simulink model "lab3_main"  (R2023a)
settings: Solver=VariableStepAuto  StartTime=0.0  StopTime=10.0  RelTol=1e-3
model workspace (MAT data in the model file):
  target = 0.05
values from neighbouring files (symbols this model uses):
  anum = 0.3    [lab3.m]
  den = [1 0 w0^2]    [lab3.m]
  denD = cell2mat(denD)    [lab3.m]
  num = G*w0^2    (= 4)    [lab3.m]
  numD = cell2mat(numD)    [lab3.m]
  Ts = 0.1    [lab3.m]
settings Model: Creator=dgkegkas2023  LastModifiedBy=dgkegkas2023

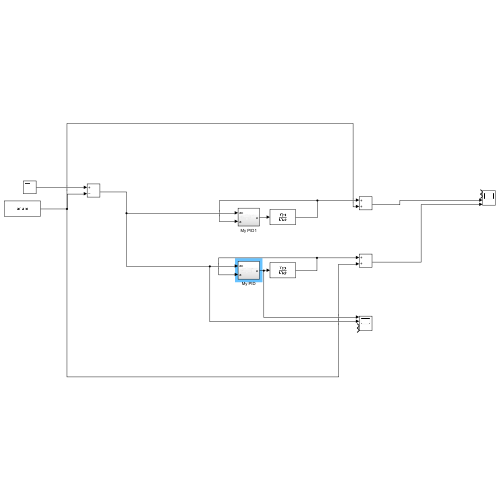
[thumbnail: Simulink's stored preview of the top-level diagram]
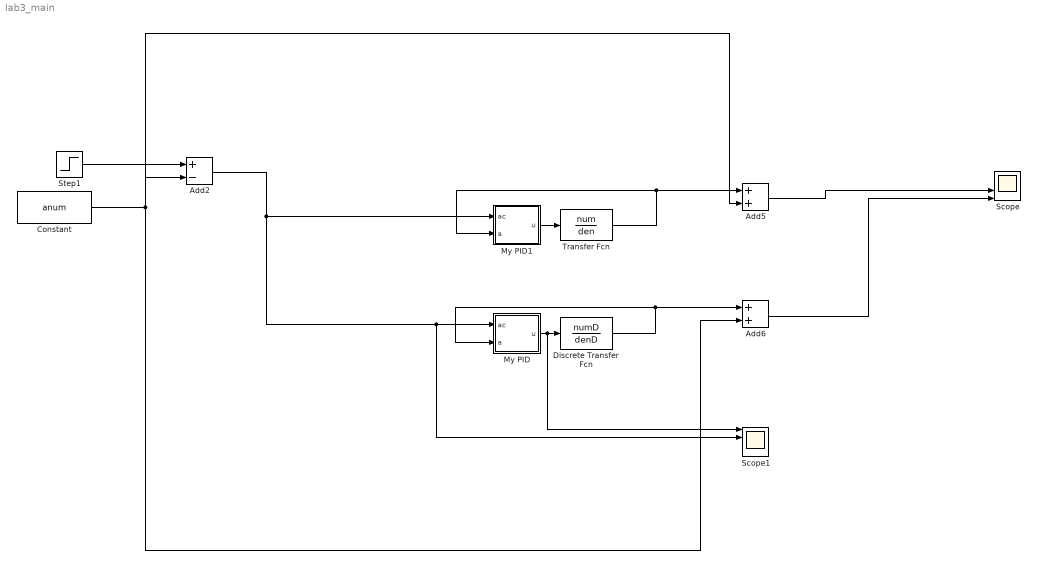
== system lab3_main ==
  Add2 : Sum  Inputs=+-
  Add5 : Sum
  Add6 : Sum
  Constant : Constant  Value=anum
  Discrete Transfer Fcn : DiscreteTransferFcn  Numerator=numD  Denominator=denD
  My PID : Subsystem
  My PID1 : Subsystem
  Scope : Scope  NumInputPorts=4
  Scope1 : Scope  NumInputPorts=4
  Step1 : Step  Before=0.3  After=0.27  SampleTime=Ts
  Transfer Fcn : TransferFcn  Numerator=num  Denominator=den
  wires:
  Transfer Fcn/1 -> My PID1/2(a), Add5/1
  Discrete Transfer Fcn/1 -> My PID/2(a), Add6/1
  Step1/1 -> Add2/1
  Constant/1 -> Add6/2, Add5/2, Add2/2
  Add2/1 -> My PID1/1(ac), Scope1/2, My PID/1(ac)
  Add5/1 -> Scope/3
  Add6/1 -> Scope/4
  My PID1/1(u) -> Transfer Fcn/1
  My PID/1(u) -> Scope1/1, Discrete Transfer Fcn/1

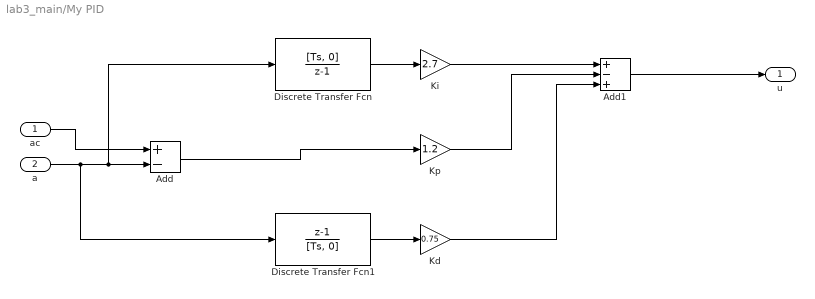
== system lab3_main/My PID ==
  ac : Inport
  a : Inport  Port=2
  Add : Sum  Inputs=+-
  Add1 : Sum  Inputs=+-+
  Discrete Transfer Fcn : DiscreteTransferFcn  Numerator=[Ts, 0]  Denominator=[1, -1]  SampleTime=Ts
  Discrete Transfer Fcn1 : DiscreteTransferFcn  Numerator=[1, -1]  Denominator=[Ts, 0]  SampleTime=Ts
  Kd : Gain  Gain=0.75
  Ki : Gain  Gain=2.7
  Kp : Gain  Gain=1.2
  u : Outport
  wires:
  ac/1 -> Add/1
  a/1 -> Discrete Transfer Fcn1/1, Discrete Transfer Fcn/1, Add/2
  Add/1 -> Kp/1
  Discrete Transfer Fcn/1 -> Ki/1
  Discrete Transfer Fcn1/1 -> Kd/1
  Kp/1 -> Add1/2
  Add1/1 -> u/1
  Ki/1 -> Add1/1
  Kd/1 -> Add1/3

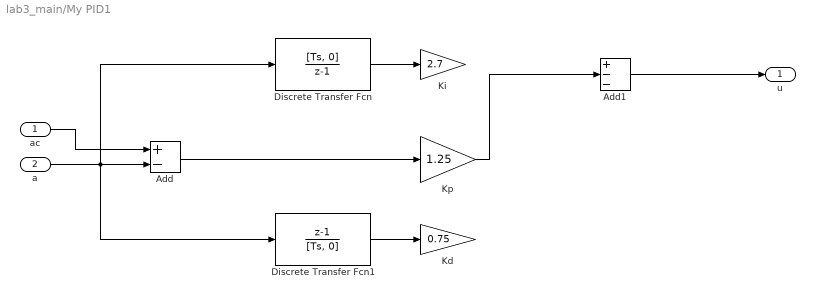
== system lab3_main/My PID1 ==
  ac : Inport
  a : Inport  Port=2
  Add : Sum  Inputs=+-
  Add1 : Sum  Inputs=+--
  Discrete Transfer Fcn : DiscreteTransferFcn  Numerator=[Ts, 0]  Denominator=[1, -1]
  Discrete Transfer Fcn1 : DiscreteTransferFcn  Numerator=[1, -1]  Denominator=[Ts, 0]
  Kd : Gain  Gain=0.75
  Ki : Gain  Gain=2.7
  Kp : Gain  Gain=1.25
  u : Outport
  wires:
  ac/1 -> Add/1
  a/1 -> Discrete Transfer Fcn/1, Add/2, Discrete Transfer Fcn1/1
  Add/1 -> Kp/1
  Discrete Transfer Fcn/1 -> Ki/1
  Discrete Transfer Fcn1/1 -> Kd/1
  Kp/1 -> Add1/2
  Add1/1 -> u/1
